simulink model "Exercitiul1"  (R2021b)
settings: Solver=VariableStepAuto  StartTime=0.0  StopTime=10.0  RelTol=1e-3

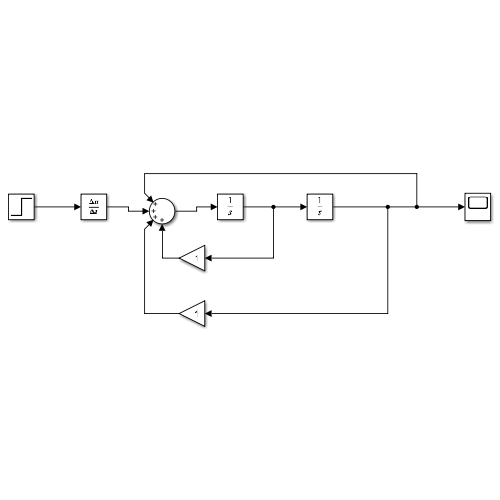
[thumbnail: Simulink's stored preview of the top-level diagram]
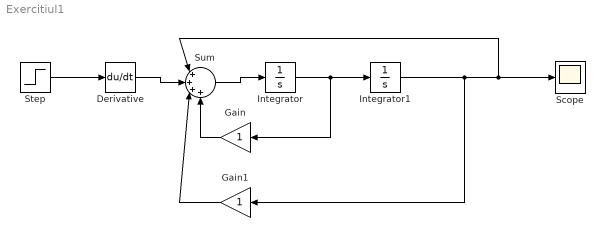
== system Exercitiul1 ==
  Derivative : Derivative
  Gain : Gain
  Gain1 : Gain
  Integrator : Integrator
  Integrator1 : Integrator
  Scope : Scope
  Step : Step  SampleTime=0
  Sum : Sum  Inputs=|++++
  wires:
  Step/1 -> Derivative/1
  Derivative/1 -> Sum/2
  Sum/1 -> Integrator/1
  Integrator/1 -> Gain/1, Integrator1/1
  Gain/1 -> Sum/4
  Gain1/1 -> Sum/3
  Integrator1/1 -> Gain1/1, Sum/1, Scope/1
